simulink library "walkingRobotUtils"  (R2017a)
settings: Solver=VariableStepAuto  StartTime=0.0  StopTime=10.0  RelTol=1e-3
undefined symbols (not defined in the file or in its folder): motion_time_constant, motor_constant, motor_inertia
undefined symbols (not defined in the file): ankle_servo_kd, ankle_servo_ki, ankle_servo_kp, deriv_filter_coeff, joint_damping, joint_stiffness, max_torque
libraries: nesl_utility x14, fl_lib x7, sm_lib x3, elec_lib x3, simulink x2, Multibody_Multiphysics_Lib x1
settings Model: Creator=scastro  LastModifiedBy=scastro

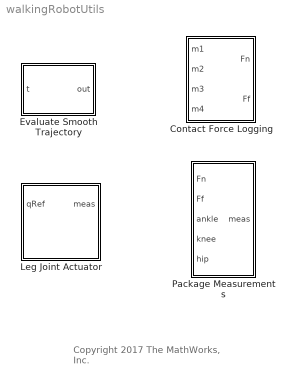
== system walkingRobotUtils ==
  note: Copyright 2017 The MathWorks, Inc.
  Contact Force Logging : Subsystem
  Evaluate Smooth Trajectory : MATLAB Function  TreatAsAtomicUnit=on
  Leg Joint Actuator : Subsystem  Variant=on  mask(Leg Joint Actuator){k=joint_stiffness, d=joint_damping, initAngle=0, Tf=motion_time_constant, Kp=ankle_servo_kp, Ki=ankle_servo_ki, Kd=ankle_servo_kd, N=deriv_filter_coeff, Tmax=max_torque}
      mask prompts: k "Joint Stiffness [N*m/rad]"; d "Joint Damping [N*m/(rad/s)]"; initAngle "Initial Joint Angle"; Tf "Motion Time Constant"; Kp "Servo Proportional Gain"; Ki "Servo Integral Gain"; Kd "Servo Derivative Gain"; N "Servo Filter Coefficient"; Tmax "Maximum Torque"
  Package Measurements : Subsystem

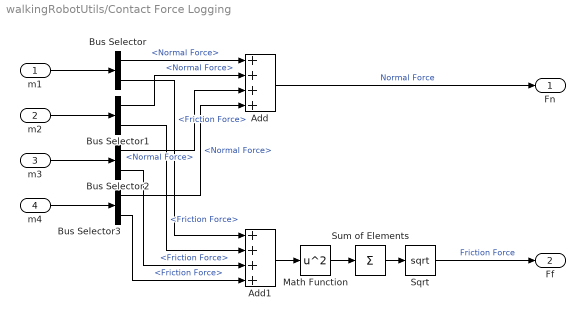
== system walkingRobotUtils/Contact Force Logging ==
  m1 : Inport
  m2 : Inport  Port=2
  m3 : Inport  Port=3
  m4 : Inport  Port=4
  Add : Sum  Inputs=4
  Add1 : Sum  Inputs=4
  Bus Selector{,1..3} (4 alike) : BusSelector  OutputSignals=Normal Force,Friction Force
  Math Function : Math  Operator=square  SaturateOnIntegerOverflow=on
  Sqrt : Sqrt  SaturateOnIntegerOverflow=on
  Sum of Elements : Sum  Inputs=+
  Fn : Outport
  Ff : Outport  Port=2
  wires:
  m1/1 -> Bus Selector/1
  m2/1 -> Bus Selector1/1
  m3/1 -> Bus Selector2/1
  m4/1 -> Bus Selector3/1
  Bus Selector/1 -> Add/1  "<Normal Force>"
  Bus Selector1/1 -> Add/2  "<Normal Force>"
  Bus Selector2/1 -> Add/3  "<Normal Force>"
  Bus Selector3/1 -> Add/4  "<Normal Force>"
  Bus Selector/2 -> Add1/1  "<Friction Force>"
  Bus Selector1/2 -> Add1/2  "<Friction Force>"
  Bus Selector2/2 -> Add1/3  "<Friction Force>"
  Bus Selector3/2 -> Add1/4  "<Friction Force>"
  Add/1 -> Fn/1  "Normal Force"
  Add1/1 -> Math Function/1
  Math Function/1 -> Sum of Elements/1
  Sum of Elements/1 -> Sqrt/1
  Sqrt/1 -> Ff/1  "Friction Force"

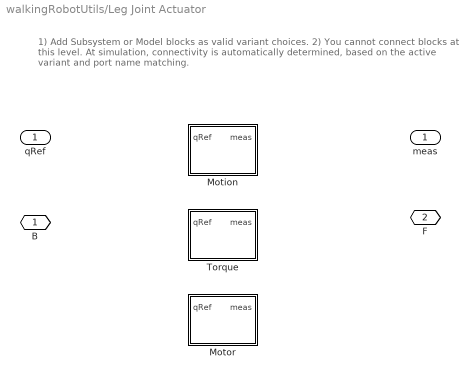
== system walkingRobotUtils/Leg Joint Actuator ==
  note: 1) Add Subsystem or Model blocks as valid variant choices.
      | 2) You cannot connect blocks at this level. At simulation, connectivity is automatically
      | determined, based on the active variant and port name matching.
  qRef : Inport
  Motion : Subsystem  VariantControl=actuatorType == 1
  Motor : Subsystem  VariantControl=actuatorType == 3
  Torque : Subsystem  VariantControl=actuatorType == 2
  B : PMIOPort  Port=1  Side=Left
  F : PMIOPort  Port=2  Side=Right
  meas : Outport

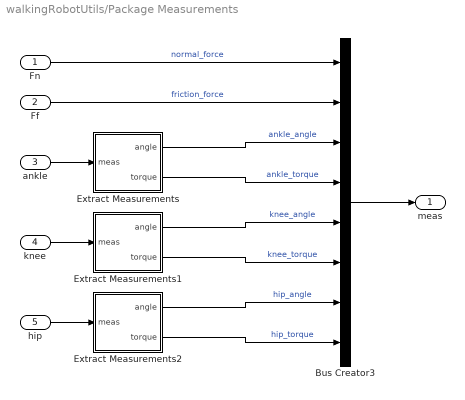
== system walkingRobotUtils/Package Measurements ==
  Fn : Inport
  Ff : Inport  Port=2
  ankle : Inport  Port=3
  knee : Inport  Port=4
  hip : Inport  Port=5
  Bus Creator3 : BusCreator  Inputs=8
  Extract Measurements : Subsystem
  Extract Measurements1 : Subsystem
  Extract Measurements2 : Subsystem
  meas : Outport
  wires:
  Bus Creator3/1 -> meas/1
  ankle/1 -> Extract Measurements/1(meas)
  Extract Measurements/1(angle) -> Bus Creator3/3  "ankle_angle"
  Extract Measurements/2(torque) -> Bus Creator3/4  "ankle_torque"
  knee/1 -> Extract Measurements1/1(meas)
  hip/1 -> Extract Measurements2/1(meas)
  Extract Measurements1/1(angle) -> Bus Creator3/5  "knee_angle"
  Extract Measurements1/2(torque) -> Bus Creator3/6  "knee_torque"
  Extract Measurements2/1(angle) -> Bus Creator3/7  "hip_angle"
  Extract Measurements2/2(torque) -> Bus Creator3/8  "hip_torque"
  Ff/1 -> Bus Creator3/2  "friction_force"
  Fn/1 -> Bus Creator3/1  "normal_force"

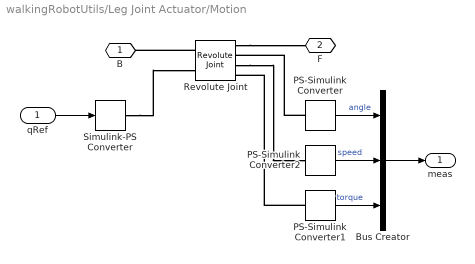
== system walkingRobotUtils/Leg Joint Actuator/Motion ==
  qRef : Inport
  Bus Creator : BusCreator  Inputs=3
  PS-Simulink Converter : nesl_utility/PS-Simulink Converter  PhysicalDomain=network_engine_domain  SubClassName=ps_output  LeftPortType=input  RightPortType=output  PseudoPeriodic=off  Frequencies=[]  Unit=deg  AffineConversion=off
  PS-Simulink Converter1 : nesl_utility/PS-Simulink Converter  PhysicalDomain=network_engine_domain  SubClassName=ps_output  LeftPortType=input  RightPortType=output  PseudoPeriodic=off  Frequencies=[]  Unit=N*m  AffineConversion=off
  PS-Simulink Converter2 : nesl_utility/PS-Simulink Converter  PhysicalDomain=network_engine_domain  SubClassName=ps_output  LeftPortType=input  RightPortType=output  PseudoPeriodic=off  Frequencies=[]  Unit=rad/s  AffineConversion=off
  Revolute Joint : sm_lib/Joints/Revolute Joint  SenseConstraintForce=off  SenseConstraintForceX=off  SenseConstraintForceY=off  SenseConstraintForceZ=off  SenseConstraintTorque=off  SenseConstraintTorqueX=off  SenseConstraintTorqueY=off  SenseConstraintTorqueZ=off  SenseTotalForce=off  SenseTotalForceX=off  SenseTotalForceY=off  SenseTotalForceZ=off  SenseTotalTorque=off  SenseTotalTorqueX=off  SenseTotalTorqueY=off  SenseTotalTorqueZ=off  CompositeWrenchDir=FollowerOnBase  CompositeWrenchFrame=BaseFrame  EquilibriumPosition=0  EquilibriumPositionUnits=deg  SpringStiffness=k  SpringStiffnessUnits=N*m/rad  DampingCoefficient=d  DampingCoefficientUnits=N*m/(rad/s)  TorqueActuationMode=ComputedTorque  MotionActuationMode=InputMotion  SensePosition=on  SenseVelocity=on  SenseAcceleration=off  SenseTorqueForce=on  PositionTargetSpecify=off  PositionTargetPriority=High  PositionTargetValue=0  PositionTargetValueUnits=rad  VelocityTargetSpecify=off  VelocityTargetPriority=High  VelocityTargetValue=0  VelocityTargetValueUnits=deg/s
  Simulink-PS Converter : nesl_utility/Simulink-PS Converter  PhysicalDomain=network_engine_domain  SubClassName=ps_input  LeftPortType=input  RightPortType=output  PseudoPeriodic=off  Frequencies=[]  NoiseDistribution=none  NoiseParameters=[]  Unit=rad  AffineConversion=off  FilteringAndDerivatives=filter  SimscapeFilterOrder=2  InputFilterTimeConstant=Tf  UdotUserProvided=0
  B : PMIOPort  Port=1  Side=Left
  F : PMIOPort  Port=2  Side=Right
  meas : Outport
  wires:
  qRef/1 -> Simulink-PS Converter/1
  PS-Simulink Converter/1 -> Bus Creator/1  "angle"
  PS-Simulink Converter1/1 -> Bus Creator/3  "torque"
  Bus Creator/1 -> meas/1
  PS-Simulink Converter2/1 -> Bus Creator/2  "speed"
  connections:
  Revolute Joint/RConn1 -- F/RConn1
  Revolute Joint/LConn1 -- B/RConn1
  Simulink-PS Converter/RConn1 -- Revolute Joint/LConn2
  PS-Simulink Converter/LConn1 -- Revolute Joint/RConn2
  PS-Simulink Converter1/LConn1 -- Revolute Joint/RConn4
  Revolute Joint/RConn3 -- PS-Simulink Converter2/LConn1

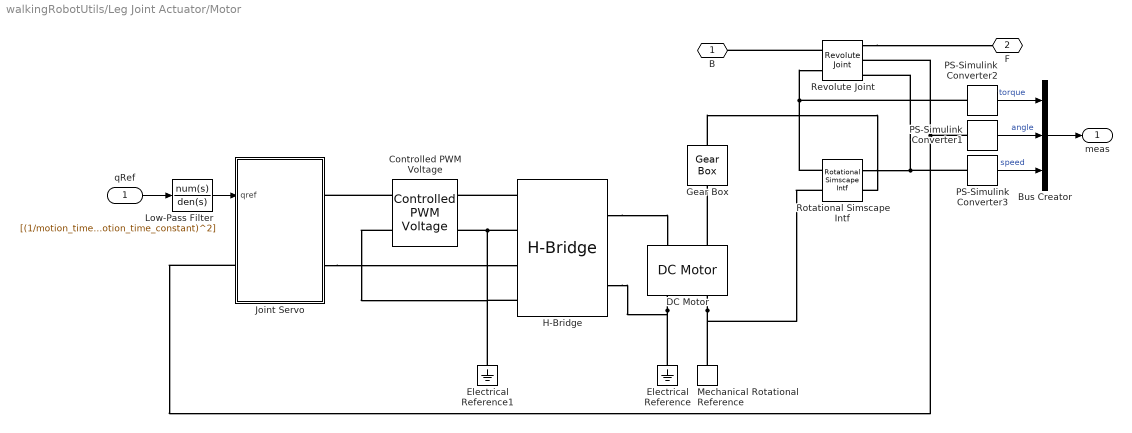
== system walkingRobotUtils/Leg Joint Actuator/Motor ==
  qRef : Inport
  Bus Creator : BusCreator  Inputs=3
  Controlled PWM Voltage : elec_lib/Actuators & Drivers/Drivers/Controlled PWM Voltage  F=1000 Hz  TD=0 s  pulse_width_offset=0 s  Vmin=0 V  Vmax=20 V  Vm=5 V  pwm_or_av=2  event_type=1  sample_time=1e-6 s
      settings: SourceProductName=Simscape Electronics  SourceProductBaseCode=SN
  DC Motor : elec_lib/Actuators & Drivers/Rotational Actuators/DC Motor  parameterization=1  Ra=motor_resistance Ohm  La=motor_inductance H  emf_or_torque=2  Kv=0.01 V/rpm  Ki=motor_constant N*m/A  T_stall=2.4e-4 N*m  w_max=1.91e+4 rpm  w_rated=1.5e+4 rpm  P_rated=0.08 W  V_rated=1.5 V  J=motor_inertia kg*m^2  lam_param=1  lam=motor_damping N*m/(rad/s)  i_noload=0 A  V_i_noload=1.5 V  speed0=0 rpm  alpha=0.00393 1/K  Tmeas=25 degC  thermal_mass=100 J/K  initial_temperature=25 degC
  Electrical Reference : fl_lib/Electrical/Electrical Elements/Electrical Reference
  Electrical Reference1 : fl_lib/Electrical/Electrical Elements/Electrical Reference
  Gear Box : fl_lib/Mechanical/Mechanisms/Gear Box  ratio=gear_ratio  t_in_specify=off  t_in_priority=None  t_in=0 N*m  t_in_nominal_specify=off  t_in_nominal_unit=N*m  t_in_nominal_value=1  t_out_specify=off  t_out_priority=None  t_out=0 N*m  t_out_nominal_specify=off  t_out_nominal_unit=N*m  t_out_nominal_value=1
  H-Bridge : elec_lib/Actuators & Drivers/Drivers/H-Bridge  Venable=1e-3 V  Vmax=5 V  Vreverse=2.5 V  Vbrake=2.5 V  Vm=24 V  pwm_or_av=2  discontinuous=0  freewheeling_mode=1  freewheeling_mode_disc=1  Ron=1e-3 Ohm  Don=1e-3 Ohm  Rload=10 Ohm  Lload=1e-5 H  F=10 kHz  thermal_mass=100 J/K  initial_temperature=298.15 K  Ron2=0.1 Ohm  Don2=0.05 Ohm  Tmeas=298.15 K  Tmeas2=398.15 K
      settings: SourceProductName=Simscape Electronics  SourceProductBaseCode=SN
  Joint Servo : Subsystem
  Low-Pass Filter : TransferFcn  Numerator=[(1/motion_time_constant)^2]  Denominator=[1 2/motion_time_constant (1/motion_time_constant)^2]
  Mechanical Rotational Reference : fl_lib/Mechanical/Rotational Elements/Mechanical Rotational Reference
  PS-Simulink Converter1 : nesl_utility/PS-Simulink Converter  PhysicalDomain=network_engine_domain  SubClassName=ps_output  LeftPortType=input  RightPortType=output  PseudoPeriodic=off  Frequencies=[]  Unit=deg  AffineConversion=off
  PS-Simulink Converter2 : nesl_utility/PS-Simulink Converter  PhysicalDomain=network_engine_domain  SubClassName=ps_output  LeftPortType=input  RightPortType=output  PseudoPeriodic=off  Frequencies=[]  Unit=N*m  AffineConversion=off
  PS-Simulink Converter3 : nesl_utility/PS-Simulink Converter  PhysicalDomain=network_engine_domain  SubClassName=ps_output  LeftPortType=input  RightPortType=output  PseudoPeriodic=off  Frequencies=[]  Unit=rad/s  AffineConversion=off
  Revolute Joint : sm_lib/Joints/Revolute Joint  SenseConstraintForce=off  SenseConstraintForceX=off  SenseConstraintForceY=off  SenseConstraintForceZ=off  SenseConstraintTorque=off  SenseConstraintTorqueX=off  SenseConstraintTorqueY=off  SenseConstraintTorqueZ=off  SenseTotalForce=off  SenseTotalForceX=off  SenseTotalForceY=off  SenseTotalForceZ=off  SenseTotalTorque=off  SenseTotalTorqueX=off  SenseTotalTorqueY=off  SenseTotalTorqueZ=off  CompositeWrenchDir=FollowerOnBase  CompositeWrenchFrame=BaseFrame  EquilibriumPosition=0  EquilibriumPositionUnits=deg  SpringStiffness=k  SpringStiffnessUnits=N*m/rad  DampingCoefficient=d  DampingCoefficientUnits=N*m/(rad/s)  TorqueActuationMode=InputTorque  MotionActuationMode=ComputedMotion  SensePosition=on  SenseVelocity=on  SenseAcceleration=off  SenseTorqueForce=off  PositionTargetSpecify=on  PositionTargetPriority=High  PositionTargetValue=initAngle  PositionTargetValueUnits=rad  VelocityTargetSpecify=off  VelocityTargetPriority=High  VelocityTargetValue=0  VelocityTargetValueUnits=deg/s
  Rotational Simscape Intf : Multibody_Multiphysics_Lib/Interfaces/Rotational Simscape Intf
      settings: SourceProductName=Simscape Multibody Multiphysics Library
  B : PMIOPort  Port=1  Side=Left
  F : PMIOPort  Port=2  Side=Right
  meas : Outport
  wires:
  Low-Pass Filter/1 -> Joint Servo/1(qref)
  qRef/1 -> Low-Pass Filter/1
  PS-Simulink Converter2/1 -> Bus Creator/1  "torque"
  Bus Creator/1 -> meas/1
  PS-Simulink Converter1/1 -> Bus Creator/2  "angle"
  PS-Simulink Converter3/1 -> Bus Creator/3  "speed"
  connections:
  DC Motor/LConn2 -- Gear Box/LConn1
  H-Bridge/RConn1 -- DC Motor/LConn1
  Joint Servo/RConn2 -- H-Bridge/LConn3
  Rotational Simscape Intf/RConn1 -- Revolute Joint/RConn3 -- PS-Simulink Converter3/LConn1
  DC Motor/RConn1 -- H-Bridge/RConn2 -- Electrical Reference/LConn1
  Controlled PWM Voltage/LConn1 -- Joint Servo/RConn1
  H-Bridge/LConn1 -- Controlled PWM Voltage/RConn1
  H-Bridge/LConn2 -- Controlled PWM Voltage/RConn2 -- Controlled PWM Voltage/LConn2 -- H-Bridge/LConn4 -- Electrical Reference1/LConn1
  Gear Box/RConn1 -- Rotational Simscape Intf/RConn2
  DC Motor/RConn2 -- Rotational Simscape Intf/LConn2 -- Mechanical Rotational Reference/LConn1
  Joint Servo/LConn1 -- Revolute Joint/RConn2 -- PS-Simulink Converter1/LConn1
  Revolute Joint/LConn1 -- B/RConn1
  Revolute Joint/RConn1 -- F/RConn1
  Rotational Simscape Intf/LConn1 -- Revolute Joint/LConn2 -- PS-Simulink Converter2/LConn1

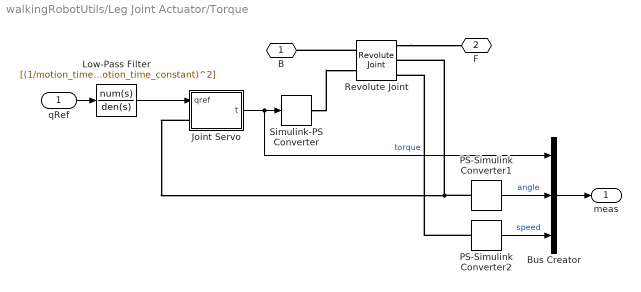
== system walkingRobotUtils/Leg Joint Actuator/Torque ==
  qRef : Inport
  Bus Creator : BusCreator  Inputs=3
  Joint Servo : Subsystem
  Low-Pass Filter : TransferFcn  Numerator=[(1/motion_time_constant)^2]  Denominator=[1 2/motion_time_constant (1/motion_time_constant)^2]
  PS-Simulink Converter1 : nesl_utility/PS-Simulink Converter  PhysicalDomain=network_engine_domain  SubClassName=ps_output  LeftPortType=input  RightPortType=output  PseudoPeriodic=off  Frequencies=[]  Unit=deg  AffineConversion=off
  PS-Simulink Converter2 : nesl_utility/PS-Simulink Converter  PhysicalDomain=network_engine_domain  SubClassName=ps_output  LeftPortType=input  RightPortType=output  PseudoPeriodic=off  Frequencies=[]  Unit=rad/s  AffineConversion=off
  Revolute Joint : sm_lib/Joints/Revolute Joint  SenseConstraintForce=off  SenseConstraintForceX=off  SenseConstraintForceY=off  SenseConstraintForceZ=off  SenseConstraintTorque=off  SenseConstraintTorqueX=off  SenseConstraintTorqueY=off  SenseConstraintTorqueZ=off  SenseTotalForce=off  SenseTotalForceX=off  SenseTotalForceY=off  SenseTotalForceZ=off  SenseTotalTorque=off  SenseTotalTorqueX=off  SenseTotalTorqueY=off  SenseTotalTorqueZ=off  CompositeWrenchDir=FollowerOnBase  CompositeWrenchFrame=BaseFrame  EquilibriumPosition=0  EquilibriumPositionUnits=deg  SpringStiffness=k  SpringStiffnessUnits=N*m/rad  DampingCoefficient=d  DampingCoefficientUnits=N*m/(rad/s)  TorqueActuationMode=InputTorque  MotionActuationMode=ComputedMotion  SensePosition=on  SenseVelocity=on  SenseAcceleration=off  SenseTorqueForce=off  PositionTargetSpecify=on  PositionTargetPriority=High  PositionTargetValue=initAngle  PositionTargetValueUnits=rad  VelocityTargetSpecify=off  VelocityTargetPriority=High  VelocityTargetValue=0  VelocityTargetValueUnits=deg/s
  Simulink-PS Converter : nesl_utility/Simulink-PS Converter  PhysicalDomain=network_engine_domain  SubClassName=ps_input  LeftPortType=input  RightPortType=output  PseudoPeriodic=off  Frequencies=[]  NoiseDistribution=none  NoiseParameters=[]  Unit=N*m  AffineConversion=off  FilteringAndDerivatives=provide  SimscapeFilterOrder=2  InputFilterTimeConstant=motion_time_constant  UdotUserProvided=0
  B : PMIOPort  Port=1  Side=Left
  F : PMIOPort  Port=2  Side=Right
  meas : Outport
  wires:
  qRef/1 -> Low-Pass Filter/1
  Low-Pass Filter/1 -> Joint Servo/1(qref)
  PS-Simulink Converter1/1 -> Bus Creator/2  "angle"
  Bus Creator/1 -> meas/1
  Joint Servo/1(t) -> Bus Creator/1, Simulink-PS Converter/1  "torque"
  PS-Simulink Converter2/1 -> Bus Creator/3  "speed"
  connections:
  Joint Servo/LConn1 -- Revolute Joint/RConn2 -- PS-Simulink Converter1/LConn1
  Revolute Joint/LConn1 -- B/RConn1
  Revolute Joint/RConn1 -- F/RConn1
  Simulink-PS Converter/RConn1 -- Revolute Joint/LConn2
  PS-Simulink Converter2/LConn1 -- Revolute Joint/RConn3

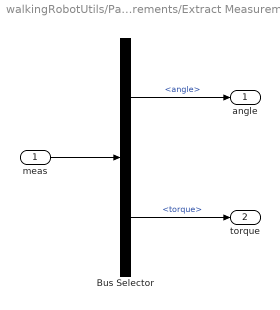
== system walkingRobotUtils/Package Measurements/Extract Measurements ==
  meas : Inport
  Bus Selector : BusSelector  OutputSignals=angle,torque
  angle : Outport
  torque : Outport  Port=2
  wires:
  Bus Selector/2 -> torque/1  "<torque>"
  meas/1 -> Bus Selector/1
  Bus Selector/1 -> angle/1  "<angle>"

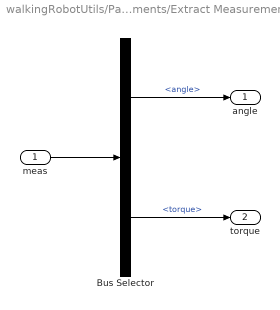
== system walkingRobotUtils/Package Measurements/Extract Measurements1 ==
  meas : Inport
  Bus Selector : BusSelector  OutputSignals=angle,torque
  angle : Outport
  torque : Outport  Port=2
  wires:
  Bus Selector/1 -> angle/1  "<angle>"
  meas/1 -> Bus Selector/1
  Bus Selector/2 -> torque/1  "<torque>"

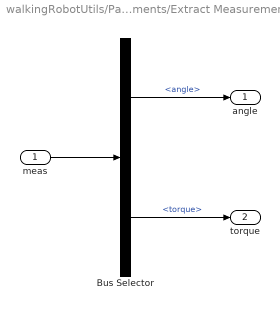
== system walkingRobotUtils/Package Measurements/Extract Measurements2 ==
  meas : Inport
  Bus Selector : BusSelector  OutputSignals=angle,torque
  angle : Outport
  torque : Outport  Port=2
  wires:
  Bus Selector/2 -> torque/1  "<torque>"
  meas/1 -> Bus Selector/1
  Bus Selector/1 -> angle/1  "<angle>"

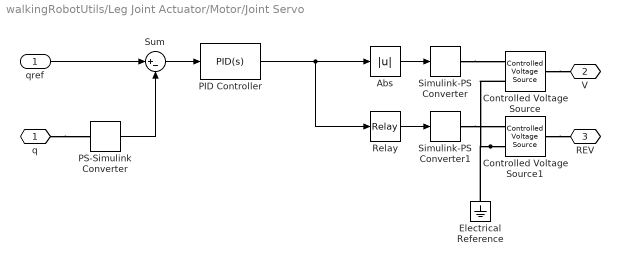
== system walkingRobotUtils/Leg Joint Actuator/Motor/Joint Servo ==
  qref : Inport
  Abs : Abs
  Controlled Voltage Source : fl_lib/Electrical/Electrical Sources/Controlled Voltage Source
  Controlled Voltage Source1 : fl_lib/Electrical/Electrical Sources/Controlled Voltage Source
  Electrical Reference : fl_lib/Electrical/Electrical Elements/Electrical Reference
  PID Controller : simulink/Continuous/PID Controller  Controller=PID  TimeDomain=Continuous-time  SampleTime=-1  IntegratorMethod=Forward Euler  FilterMethod=Forward Euler  Form=Parallel  UseFilter=on  ControllerParametersSource=internal  P=Kp  I=Ki  D=Kd  N=N  InitialConditionSource=internal  InitialConditionForIntegrator=0  InitialConditionForFilter=0  ExternalReset=none  ZeroCross=off  LimitOutput=on  UpperSaturationLimit=Tmax  LowerSaturationLimit=-Tmax  LinearizeAsGain=on  AntiWindupMode=clamping  Kb=1  TrackingMode=off  Kt=1  PParamMin=[]  PParamMax=[]  IParamMin=[]  IParamMax=[]  DParamMin=[]  DParamMax=[]  NParamMin=[]  NParamMax=[]  KbParamMin=[]  KbParamMax=[]  KtParamMin=[]  KtParamMax=[]  POutMin=[]  POutMax=[]  IOutMin=[]  IOutMax=[]  DOutMin=[]  DOutMax=[]  NOutMin=[]  NOutMax=[]  KbOutMin=[]  KbOutMax=[]  KtOutMin=[]  KtOutMax=[]  IntegratorOutMin=[]  IntegratorOutMax=[]  FilterOutMin=[]  FilterOutMax=[]  SumOutMin=[]  SumOutMax=[]  SumI1OutMin=[]  SumI1OutMax=[]  SumI2OutMin=[]  SumI2OutMax=[]  SumI3OutMin=[]  SumI3OutMax=[]  SumDOutMin=[]  SumDOutMax=[]  SaturationOutMin=[]  SaturationOutMax=[]  IntegratorContinuousStateAttributes=''  IntegratorStateMustResolveToSignalObject=off  IntegratorRTWStateStorageClass=Auto  FilterContinuousStateAttributes=''  FilterStateMustResolveToSignalObject=off  FilterRTWStateStorageClass=Auto  DifferentiatorICPrevScaledInput=0  DifferentiatorOutMin=[]  DifferentiatorOutMax=[]  InitialConditionSetting=State (most efficient)
  PS-Simulink Converter : nesl_utility/PS-Simulink Converter  PhysicalDomain=network_engine_domain  SubClassName=ps_output  LeftPortType=input  RightPortType=output  PseudoPeriodic=off  Frequencies=[]  Unit=rad  AffineConversion=off
  Relay : Relay  OnSwitchValue=1e-3  OffSwitchValue=-1e-3  OnOutputValue=0  OffOutputValue=5
  Simulink-PS Converter : nesl_utility/Simulink-PS Converter  PhysicalDomain=network_engine_domain  SubClassName=ps_input  LeftPortType=input  RightPortType=output  PseudoPeriodic=off  Frequencies=[]  NoiseDistribution=none  NoiseParameters=[]  Unit=1  AffineConversion=off  FilteringAndDerivatives=provide  SimscapeFilterOrder=1  InputFilterTimeConstant=0.005  UdotUserProvided=0
  Simulink-PS Converter1 : nesl_utility/Simulink-PS Converter  PhysicalDomain=network_engine_domain  SubClassName=ps_input  LeftPortType=input  RightPortType=output  PseudoPeriodic=off  Frequencies=[]  NoiseDistribution=none  NoiseParameters=[]  Unit=1  AffineConversion=off  FilteringAndDerivatives=provide  SimscapeFilterOrder=1  InputFilterTimeConstant=0.005  UdotUserProvided=0
  Sum : Sum  Inputs=|+-
  q : PMIOPort  Port=1  Side=Left
  V : PMIOPort  Port=2  Side=Right
  REV : PMIOPort  Port=3  Side=Right
  wires:
  Relay/1 -> Simulink-PS Converter1/1
  Abs/1 -> Simulink-PS Converter/1
  Sum/1 -> PID Controller/1
  PS-Simulink Converter/1 -> Sum/2
  qref/1 -> Sum/1
  PID Controller/1 -> Relay/1, Abs/1
  connections:
  Simulink-PS Converter1/RConn1 -- Controlled Voltage Source1/RConn1
  Controlled Voltage Source1/LConn1 -- REV/RConn1
  Controlled Voltage Source1/RConn2 -- Controlled Voltage Source/RConn2 -- Electrical Reference/LConn1
  Controlled Voltage Source/LConn1 -- V/RConn1
  Simulink-PS Converter/RConn1 -- Controlled Voltage Source/RConn1
  q/RConn1 -- PS-Simulink Converter/LConn1

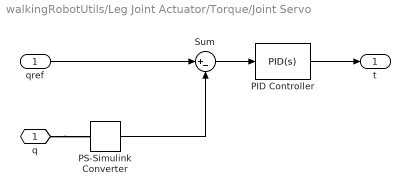
== system walkingRobotUtils/Leg Joint Actuator/Torque/Joint Servo ==
  qref : Inport
  PID Controller : simulink/Continuous/PID Controller  Controller=PID  TimeDomain=Continuous-time  SampleTime=-1  IntegratorMethod=Forward Euler  FilterMethod=Forward Euler  Form=Parallel  UseFilter=on  ControllerParametersSource=internal  P=Kp  I=Ki  D=Kd  N=N  InitialConditionSource=internal  InitialConditionForIntegrator=0  InitialConditionForFilter=0  ExternalReset=none  ZeroCross=off  LimitOutput=on  UpperSaturationLimit=Tmax  LowerSaturationLimit=-Tmax  LinearizeAsGain=on  AntiWindupMode=clamping  Kb=1  TrackingMode=off  Kt=1  PParamMin=[]  PParamMax=[]  IParamMin=[]  IParamMax=[]  DParamMin=[]  DParamMax=[]  NParamMin=[]  NParamMax=[]  KbParamMin=[]  KbParamMax=[]  KtParamMin=[]  KtParamMax=[]  POutMin=[]  POutMax=[]  IOutMin=[]  IOutMax=[]  DOutMin=[]  DOutMax=[]  NOutMin=[]  NOutMax=[]  KbOutMin=[]  KbOutMax=[]  KtOutMin=[]  KtOutMax=[]  IntegratorOutMin=[]  IntegratorOutMax=[]  FilterOutMin=[]  FilterOutMax=[]  SumOutMin=[]  SumOutMax=[]  SumI1OutMin=[]  SumI1OutMax=[]  SumI2OutMin=[]  SumI2OutMax=[]  SumI3OutMin=[]  SumI3OutMax=[]  SumDOutMin=[]  SumDOutMax=[]  SaturationOutMin=[]  SaturationOutMax=[]  IntegratorContinuousStateAttributes=''  IntegratorStateMustResolveToSignalObject=off  IntegratorRTWStateStorageClass=Auto  FilterContinuousStateAttributes=''  FilterStateMustResolveToSignalObject=off  FilterRTWStateStorageClass=Auto  DifferentiatorICPrevScaledInput=0  DifferentiatorOutMin=[]  DifferentiatorOutMax=[]  InitialConditionSetting=State (most efficient)
  PS-Simulink Converter : nesl_utility/PS-Simulink Converter  PhysicalDomain=network_engine_domain  SubClassName=ps_output  LeftPortType=input  RightPortType=output  PseudoPeriodic=off  Frequencies=[]  Unit=rad  AffineConversion=off
  Sum : Sum  Inputs=|+-
  q : PMIOPort  Port=1  Side=Left
  t : Outport
  wires:
  qref/1 -> Sum/1
  PS-Simulink Converter/1 -> Sum/2
  Sum/1 -> PID Controller/1
  PID Controller/1 -> t/1
  connections:
  q/RConn1 -- PS-Simulink Converter/LConn1

== matlab function walkingRobotUtils/Evaluate Smooth Trajectory ==
  data: t input; out output; curveData parameter
function out = smoothTraj(t,curveData)

    % Call evalSmoothTrajectory function
    out = evalSmoothTrajectory(curveData,t);

end
